simulink model "mdl_foc_platform"  (R2023a)
settings: configuration reference "cfg_FocCodeGeneration_v04" (kept outside this file)
undefined symbols (not defined in the file): Cdbl_nMechSpdPeakVal, cstPermMagTempCoef, cstPolePairNum, cstRefTemp, Gu16_rCtlBrdVltgADCRat_C, Gu16_rGDVltgADCRat_C, Gu16_rPhCurrADCRat_C, Gu16_rSplyVltgADCRat_C, Gu16_tMotoTemp_CUR_ADMotoTempADC_X, Gu16_tPCBTemp_CUR_ADPCBTempADC_X, Gu16_tPwrTubTemp_CUR_ADPwrTubTempADC_X, Gu8_tMotoTemp_CUR, Gu8_tPCBTemp_CUR, Gu8_tPwrTubTemp_CUR, parAmbPermMagFlux, parDirIndc, parPolePairNum, parQdrtIndc
libraries: lib_conversion x10, eeTransforms x1, simulink x1, lib_park_transform x1
(part 2 of 2)

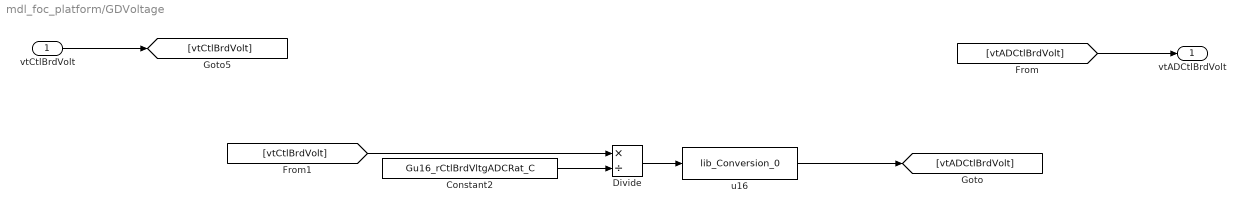
== system mdl_foc_platform/GDVoltage ==
  vtCtlBrdVolt : Inport
  Constant2 : Constant  Value=Gu16_rCtlBrdVltgADCRat_C
  Divide : Product  Inputs=*/  OutDataTypeStr=Inherit: Inherit via back propagation
  u16 : lib_conversion/lib_Conversion_0  lb_parDataType=uint16  lb_parOutpMaxVal=[]  lb_parOutpMinVal=[]  lb_parSatFlag=off
  vtADCtlBrdVolt : Outport
  wires:
  Divide/1 -> u16/1
  Constant2/1 -> Divide/2
  u16/1 -> [vtADCtlBrdVolt]
  [vtCtlBrdVolt] -> Divide/1
  [vtADCtlBrdVolt] -> vtADCtlBrdVolt/1
  vtCtlBrdVolt/1 -> [vtCtlBrdVolt]

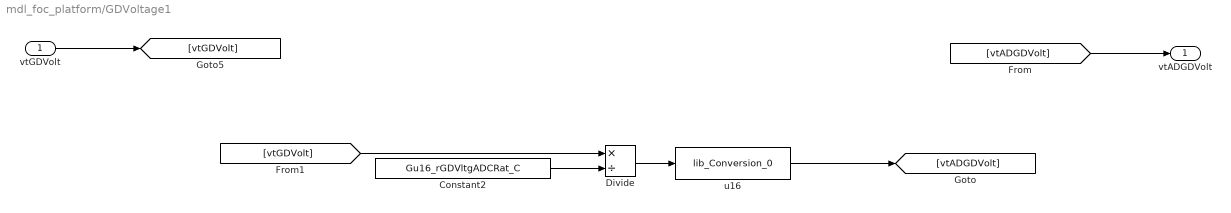
== system mdl_foc_platform/GDVoltage1 ==
  vtGDVolt : Inport
  Constant2 : Constant  Value=Gu16_rGDVltgADCRat_C
  Divide : Product  Inputs=*/  OutDataTypeStr=Inherit: Inherit via back propagation
  u16 : lib_conversion/lib_Conversion_0  lb_parDataType=uint16  lb_parOutpMaxVal=[]  lb_parOutpMinVal=[]  lb_parSatFlag=off
  vtADGDVolt : Outport
  wires:
  Divide/1 -> u16/1
  Constant2/1 -> Divide/2
  u16/1 -> [vtADGDVolt]
  [vtGDVolt] -> Divide/1
  [vtADGDVolt] -> vtADGDVolt/1
  vtGDVolt/1 -> [vtGDVolt]

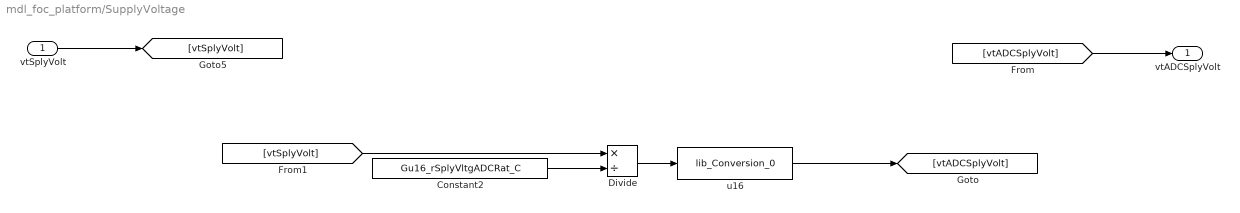
== system mdl_foc_platform/SupplyVoltage ==
  vtSplyVolt : Inport
  Constant2 : Constant  Value=Gu16_rSplyVltgADCRat_C
  Divide : Product  Inputs=*/  OutDataTypeStr=Inherit: Inherit via back propagation
  u16 : lib_conversion/lib_Conversion_0  lb_parDataType=uint16  lb_parOutpMaxVal=[]  lb_parOutpMinVal=[]  lb_parSatFlag=off
  vtADCSplyVolt : Outport
  wires:
  Divide/1 -> u16/1
  u16/1 -> [vtADCSplyVolt]
  [vtSplyVolt] -> Divide/1
  [vtADCSplyVolt] -> vtADCSplyVolt/1
  vtSplyVolt/1 -> [vtSplyVolt]
  Constant2/1 -> Divide/2

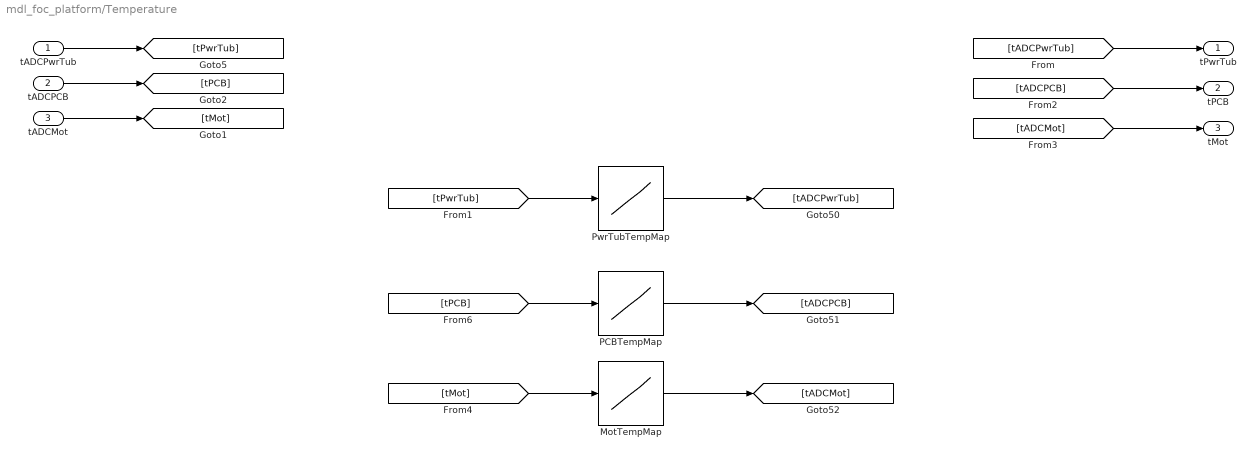
== system mdl_foc_platform/Temperature ==
  tADCPwrTub : Inport
  tADCPCB : Inport  Port=2
  tADCMot : Inport  Port=3
  MotTempMap : Lookup_n-D  NumberOfTableDimensions=1  BreakpointsForDimension1=Gu8_tMotoTemp_CUR  Table=Gu16_tMotoTemp_CUR_ADMotoTempADC_X  ExtrapMethod=Clip  InternalRulePriority=Speed  OutDataTypeStr=Inherit: Inherit from 'Table data'  RndMeth=Simplest
  PCBTempMap : Lookup_n-D  NumberOfTableDimensions=1  BreakpointsForDimension1=Gu8_tPCBTemp_CUR  Table=Gu16_tPCBTemp_CUR_ADPCBTempADC_X  ExtrapMethod=Clip  InternalRulePriority=Speed  OutDataTypeStr=Inherit: Inherit from 'Table data'  RndMeth=Simplest
  PwrTubTempMap : Lookup_n-D  NumberOfTableDimensions=1  BreakpointsForDimension1=Gu8_tPwrTubTemp_CUR  Table=Gu16_tPwrTubTemp_CUR_ADPwrTubTempADC_X  ExtrapMethod=Clip  InternalRulePriority=Speed  OutDataTypeStr=Inherit: Inherit from 'Table data'  RndMeth=Simplest
  tPwrTub : Outport
  tPCB : Outport  Port=2
  tMot : Outport  Port=3
  wires:
  tADCPwrTub/1 -> [tPwrTub]
  tADCPCB/1 -> [tPCB]
  tADCMot/1 -> [tMot]
  [tPwrTub] -> PwrTubTempMap/1
  [tPCB] -> PCBTempMap/1
  [tMot] -> MotTempMap/1
  [tADCMot] -> tMot/1
  [tADCPCB] -> tPCB/1
  [tADCPwrTub] -> tPwrTub/1
  PwrTubTempMap/1 -> [tADCPwrTub]
  PCBTempMap/1 -> [tADCPCB]
  MotTempMap/1 -> [tADCMot]

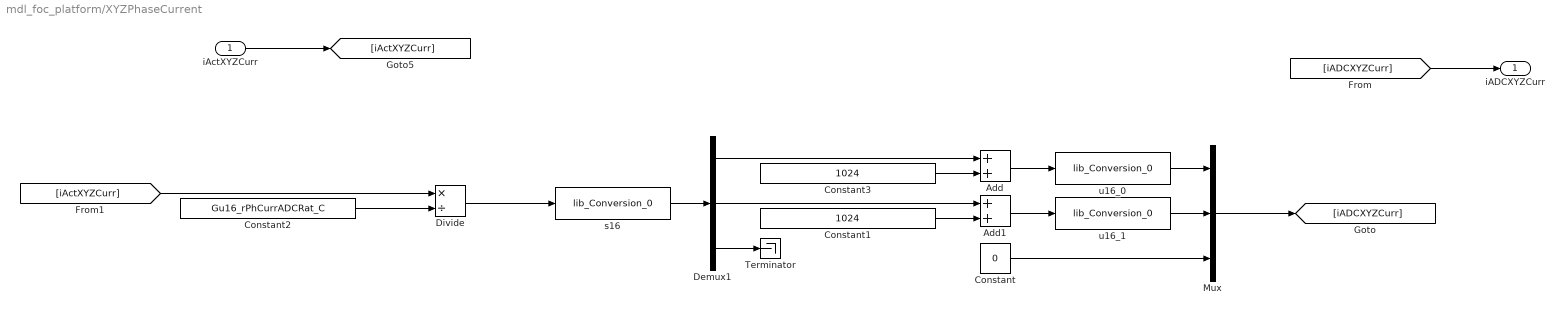
== system mdl_foc_platform/XYZPhaseCurrent ==
  iActXYZCurr : Inport
  Add : Sum  OutDataTypeStr=Inherit: Inherit via back propagation
  Add1 : Sum  OutDataTypeStr=Inherit: Inherit via back propagation
  Constant : Constant  Value=0  OutDataTypeStr=uint16
  Constant1 : Constant  Value=1024  OutDataTypeStr=int16
  Constant2 : Constant  Value=Gu16_rPhCurrADCRat_C
  Constant3 : Constant  Value=1024  OutDataTypeStr=int16
  Demux1 : Demux  Outputs=3
  Divide : Product  Inputs=*/  OutDataTypeStr=Inherit: Inherit via back propagation
  Mux : Mux  Inputs=3
  Terminator : Terminator
  s16 : lib_conversion/lib_Conversion_0  lb_parDataType=int16  lb_parOutpMaxVal=[]  lb_parOutpMinVal=[]  lb_parSatFlag=off
  u16_0 : lib_conversion/lib_Conversion_0  lb_parDataType=uint16  lb_parOutpMaxVal=[]  lb_parOutpMinVal=[]  lb_parSatFlag=off
  u16_1 : lib_conversion/lib_Conversion_0  lb_parDataType=uint16  lb_parOutpMaxVal=[]  lb_parOutpMinVal=[]  lb_parSatFlag=off
  iADCXYZCurr : Outport
  wires:
  Demux1/1 -> Add/1
  Constant3/1 -> Add/2
  Demux1/2 -> Add1/1
  Constant1/1 -> Add1/2
  Demux1/3 -> Terminator/1
  Add/1 -> u16_0/1
  Add1/1 -> u16_1/1
  Constant/1 -> Mux/3
  iActXYZCurr/1 -> [iActXYZCurr]
  [iADCXYZCurr] -> iADCXYZCurr/1
  [iActXYZCurr] -> Divide/1
  Mux/1 -> [iADCXYZCurr]
  s16/1 -> Demux1/1
  Divide/1 -> s16/1
  u16_0/1 -> Mux/1
  u16_1/1 -> Mux/2
  Constant2/1 -> Divide/2

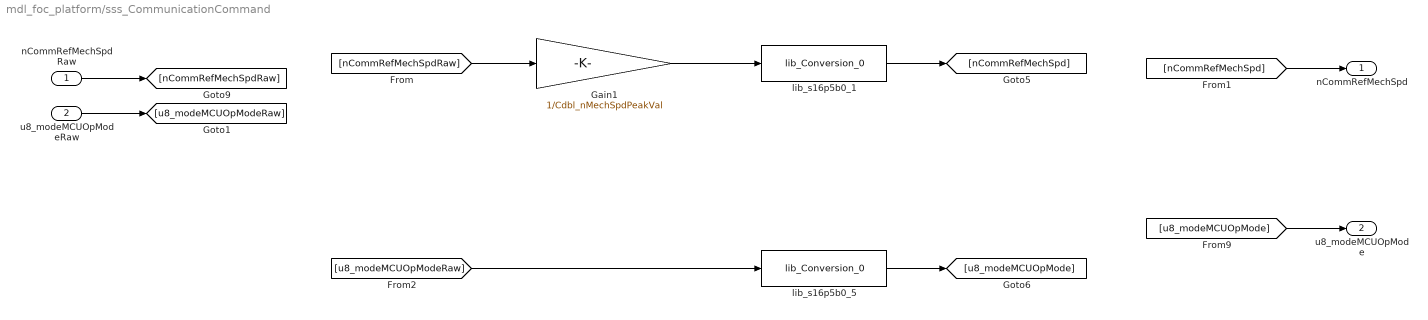
== system mdl_foc_platform/sss_CommunicationCommand ==
  nCommRefMechSpdRaw : Inport  OutDataTypeStr=int16
  u8_modeMCUOpModeRaw : Inport  Port=2  OutDataTypeStr=uint8
  Gain1 : Gain  Gain=1/Cdbl_nMechSpdPeakVal  OutDataTypeStr=Inherit: Inherit via back propagation
  lib_s16p5b0_1 : lib_conversion/lib_Conversion_0  lb_parDataType=dt_Standardize_s16p15b0  lb_parOutpMaxVal=[]  lb_parOutpMinVal=[]  lb_parSatFlag=off
  lib_s16p5b0_5 : lib_conversion/lib_Conversion_0  lb_parDataType=uint8  lb_parOutpMaxVal=[]  lb_parOutpMinVal=[]  lb_parSatFlag=off
  nCommRefMechSpd : Outport  OutDataTypeStr=dt_Standardize_s16p15b0
  u8_modeMCUOpMode : Outport  Port=2  OutDataTypeStr=uint8
  wires:
  [nCommRefMechSpd] -> nCommRefMechSpd/1
  nCommRefMechSpdRaw/1 -> [nCommRefMechSpdRaw]
  lib_s16p5b0_1/1 -> [nCommRefMechSpd]
  [nCommRefMechSpdRaw] -> Gain1/1
  [u8_modeMCUOpModeRaw] -> lib_s16p5b0_5/1
  lib_s16p5b0_5/1 -> [u8_modeMCUOpMode]
  [u8_modeMCUOpMode] -> u8_modeMCUOpMode/1
  Gain1/1 -> lib_s16p5b0_1/1
  u8_modeMCUOpModeRaw/1 -> [u8_modeMCUOpModeRaw]

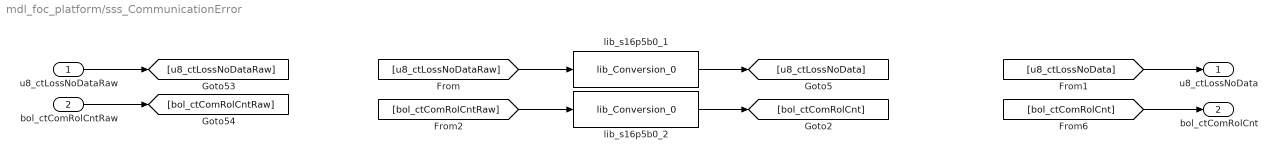
== system mdl_foc_platform/sss_CommunicationError ==
  u8_ctLossNoDataRaw : Inport  OutDataTypeStr=uint8
  bol_ctComRolCntRaw : Inport  Port=2  OutDataTypeStr=uint8
  lib_s16p5b0_1 : lib_conversion/lib_Conversion_0  lb_parDataType=uint8  lb_parOutpMaxVal=[]  lb_parOutpMinVal=[]  lb_parSatFlag=off
  lib_s16p5b0_2 : lib_conversion/lib_Conversion_0  lb_parDataType=uint8  lb_parOutpMaxVal=[]  lb_parOutpMinVal=[]  lb_parSatFlag=off
  u8_ctLossNoData : Outport  OutDataTypeStr=uint8
  bol_ctComRolCnt : Outport  Port=2  OutDataTypeStr=uint8
  wires:
  [bol_ctComRolCnt] -> bol_ctComRolCnt/1
  lib_s16p5b0_2/1 -> [bol_ctComRolCnt]
  [bol_ctComRolCntRaw] -> lib_s16p5b0_2/1
  [u8_ctLossNoDataRaw] -> lib_s16p5b0_1/1
  lib_s16p5b0_1/1 -> [u8_ctLossNoData]
  [u8_ctLossNoData] -> u8_ctLossNoData/1
  u8_ctLossNoDataRaw/1 -> [u8_ctLossNoDataRaw]
  bol_ctComRolCntRaw/1 -> [bol_ctComRolCntRaw]

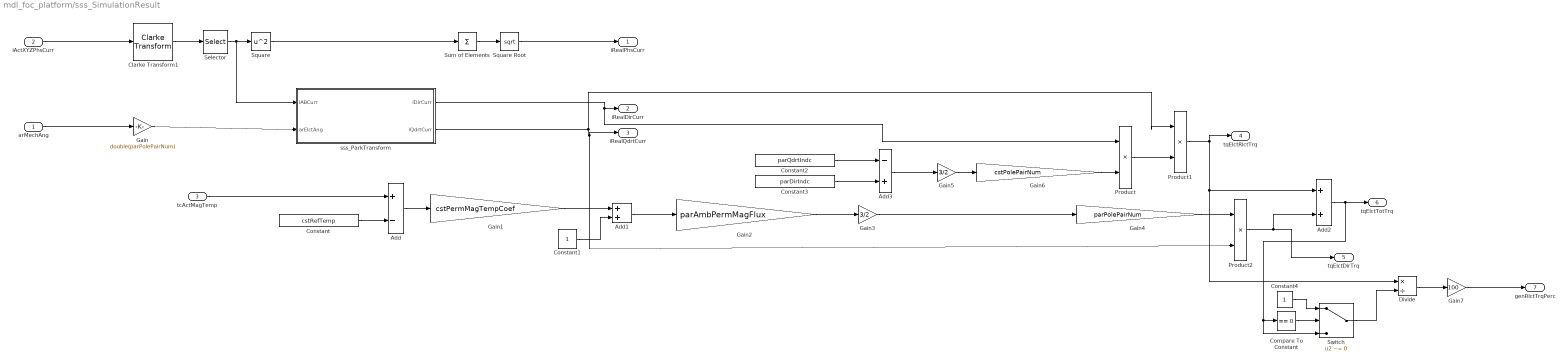
== system mdl_foc_platform/sss_SimulationResult ==
  arMechAng : Inport
  iActXYZPhsCurr : Inport  Port=2
  tcActMagTemp : Inport  Port=3
  Add : Sum  Inputs=+-
  Add1 : Sum
  Add2 : Sum
  Add3 : Sum  Inputs=-+
  Clarke Transform1 : eeTransforms/Clarke Transform  PowerInvariant=off
  Compare To Constant : simulink/Logic and Bit Operations/Compare To Constant  relop===  const=0  OutDataTypeStr=boolean
  Constant : Constant  Value=cstRefTemp  OutDataTypeStr=double
  Constant1 : Constant
  Constant2 : Constant  Value=parQdrtIndc  OutDataTypeStr=double
  Constant3 : Constant  Value=parDirIndc  OutDataTypeStr=double
  Constant4 : Constant
  Divide : Product  Inputs=*/
  Gain : Gain  Gain=double(parPolePairNum)
  Gain1 : Gain  Gain=cstPermMagTempCoef  OutDataTypeStr=double
  Gain2 : Gain  Gain=parAmbPermMagFlux  OutDataTypeStr=double
  Gain3 : Gain  Gain=3/2
  Gain4 : Gain  Gain=parPolePairNum
  Gain5 : Gain  Gain=3/2
  Gain6 : Gain  Gain=cstPolePairNum
  Gain7 : Gain  Gain=100
  Product : Product
  Product1 : Product
  Product2 : Product
  Selector : Selector  InputPortWidth=3  IndexOptions=Index vector (dialog)  Indices=[1 2]  OutputSizes=1
  Square : Math  Operator=square
  Square Root : Sqrt
  Sum of Elements : Sum  Inputs=+
  Switch : Switch  Criteria=u2 ~= 0  SaturateOnIntegerOverflow=off  InputSameDT=off
  sss_ParkTransform : Subsystem
  iRealPhsCurr : Outport
  iRealDirCurr : Outport  Port=2
  iRealQdrtCurr : Outport  Port=3
  tqElctRlctTrq : Outport  Port=4
  tqElctDirTrq : Outport  Port=5
  tqElctTotTrq : Outport  Port=6
  genRlctTrqPerc : Outport  Port=7
  wires:
  Selector/1 -> sss_ParkTransform/1(iABCurr), Square/1
  Clarke Transform1/1 -> Selector/1
  Square/1 -> Sum of Elements/1
  Sum of Elements/1 -> Square Root/1
  Square Root/1 -> iRealPhsCurr/1
  iActXYZPhsCurr/1 -> Clarke Transform1/1
  arMechAng/1 -> Gain/1
  sss_ParkTransform/1(iDirCurr) -> Product/1, iRealDirCurr/1
  sss_ParkTransform/2(iQdrtCurr) -> Product2/2, iRealQdrtCurr/1, Product1/1
  tcActMagTemp/1 -> Add/1
  Constant/1 -> Add/2
  Add/1 -> Gain1/1
  Gain1/1 -> Add1/1
  Constant1/1 -> Add1/2
  Add1/1 -> Gain2/1
  Gain3/1 -> Gain4/1
  Gain2/1 -> Gain3/1
  Constant2/1 -> Add3/1
  Constant3/1 -> Add3/2
  Add2/1 -> Switch/3, Compare To Constant/1, tqElctTotTrq/1
  Product/1 -> Product1/2
  Product1/1 -> Divide/1, Add2/1, tqElctRlctTrq/1
  Gain4/1 -> Product2/1
  Product2/1 -> Add2/2, tqElctDirTrq/1
  Add3/1 -> Gain5/1
  Gain5/1 -> Gain6/1
  Gain6/1 -> Product/2
  Divide/1 -> Gain7/1
  Gain7/1 -> genRlctTrqPerc/1
  Compare To Constant/1 -> Switch/2
  Constant4/1 -> Switch/1
  Switch/1 -> Divide/2
  Gain/1 -> sss_ParkTransform/2(arElctAng)

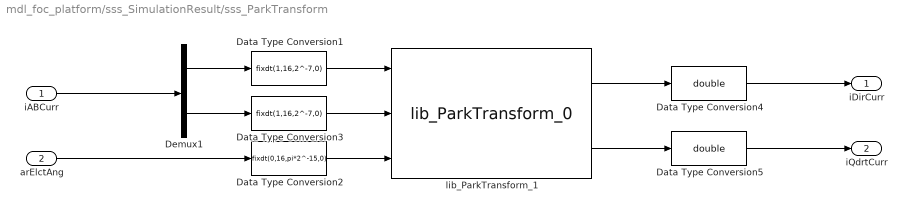
== system mdl_foc_platform/sss_SimulationResult/sss_ParkTransform ==
  iABCurr : Inport
  arElctAng : Inport  Port=2
  Data Type Conversion1 : DataTypeConversion  OutDataTypeStr=fixdt(1,16,2^-7,0)  SaturateOnIntegerOverflow=off  RndMeth=Floor
  Data Type Conversion2 : DataTypeConversion  OutDataTypeStr=fixdt(0,16,pi*2^-15,0)  SaturateOnIntegerOverflow=off  RndMeth=Floor
  Data Type Conversion3 : DataTypeConversion  OutDataTypeStr=fixdt(1,16,2^-7,0)  SaturateOnIntegerOverflow=off  RndMeth=Floor
  Data Type Conversion4 : DataTypeConversion  OutDataTypeStr=double  SaturateOnIntegerOverflow=off  RndMeth=Floor
  Data Type Conversion5 : DataTypeConversion  OutDataTypeStr=double  SaturateOnIntegerOverflow=off  RndMeth=Floor
  Demux1 : Demux  Outputs=2
  lib_ParkTransform_1 : lib_park_transform/lib_ParkTransform_0  VariantControl=ClarkTransf_MIL_flo  lb_parSelRotFrmeAxis=d-axis
  iDirCurr : Outport
  iQdrtCurr : Outport  Port=2
  wires:
  Demux1/2 -> Data Type Conversion3/1
  Data Type Conversion1/1 -> lib_ParkTransform_1/1
  Demux1/1 -> Data Type Conversion1/1
  Data Type Conversion3/1 -> lib_ParkTransform_1/2
  lib_ParkTransform_1/1 -> Data Type Conversion4/1
  arElctAng/1 -> Data Type Conversion2/1
  lib_ParkTransform_1/2 -> Data Type Conversion5/1
  Data Type Conversion2/1 -> lib_ParkTransform_1/3
  Data Type Conversion4/1 -> iDirCurr/1
  iABCurr/1 -> Demux1/1
  Data Type Conversion5/1 -> iQdrtCurr/1
